simulink model "qddot"  (R2019b)
settings: Solver=ode3  StartTime=0.0  StopTime=10  FixedStep=0.001  RelTol=1e-3  EnableMultiTasking=on
settings Model: ExtModeTrigDuration=5000  Creator=sfukamachi  LastModifiedBy=Chris
settings SolverCC: PositivePriorityOrder=on
settings DataIOCC: LimitDataPoints=on  SaveFormat=Array  ReturnWorkspaceOutputs=off
settings OptimizationCC: ExpressionDepthLimit=2147483647  LifeSpan=inf
settings DebuggingCC: UnderspecifiedInitializationDetection=Classic  MergeDetectMultiDrivingBlocksExec=none  SolverPrmCheckMsg=warning  StateNameClashWarn=warning  SFUnexpectedBacktrackingDiag=warning  SFNoUnconditionalDefaultTransitionDiag=warning  SFExecutionAtInitializationDiag=none  ArithmeticOperatorsInVariantConditions=warning
settings HardwareCC: ProdBitPerPointer=32  ProdBitPerSizeT=32  ProdBitPerPtrDiffT=32  ProdLargestAtomicFloat=None  ProdIntDivRoundTo=Undefined  ProdEndianess=Unspecified  ProdWordSize=32  ProdHWDeviceType=32-bit Generic
settings ModelReferenceCC: PropagateSignalLabelsOutOfModel=off
settings SFSimCC: SimUseLocalCustomCode=off  CustomCodeUndefinedFunction=UseInterfaceOnly
settings RTWCC: Description=QUARC Win64 Target  SystemTargetFile=quarc_win64.tlc  TemplateMakefile=quarc_default_tmf  RTWUseLocalCustomCode=off
settings CodeAppCC: StateflowObjectComments=on
settings STFCustomTargetCC: TargetPreCompLibLocation=C:\PROGRA~3\QUARC\lib\2012b\win64\release  GeneratePreprocessorConditionals=Disable all  CombineOutputUpdateFcns=on  CPPClassGenCompliant=on  SystemTargetFile=quarc_win64.tlc
settings GRTTargetCC: TargetPreCompLibLocation=C:\PROGRA~3\QUARC\lib\2012b\win64\release  TargetLangStandard=C89/C90 (ANSI)  ParMdlRefBuildCompliant=off  CompOptLevelCompliant=off  ConcurrentExecutionCompliant=off  GeneratePreprocessorConditionals=Disable all  MatFileLogging=off  UseToolchainInfoCompliant=off  ExtMode=on  ExtModeMexFile=quarc_comm
settings ConfigComp: CovMetricSettings=dw  CovHtmlReporting=on  CovSaveCumulativeToWorkspaceVar=on  CovSaveSingleToWorkspaceVar=on  CovExternalEMLEnable=off

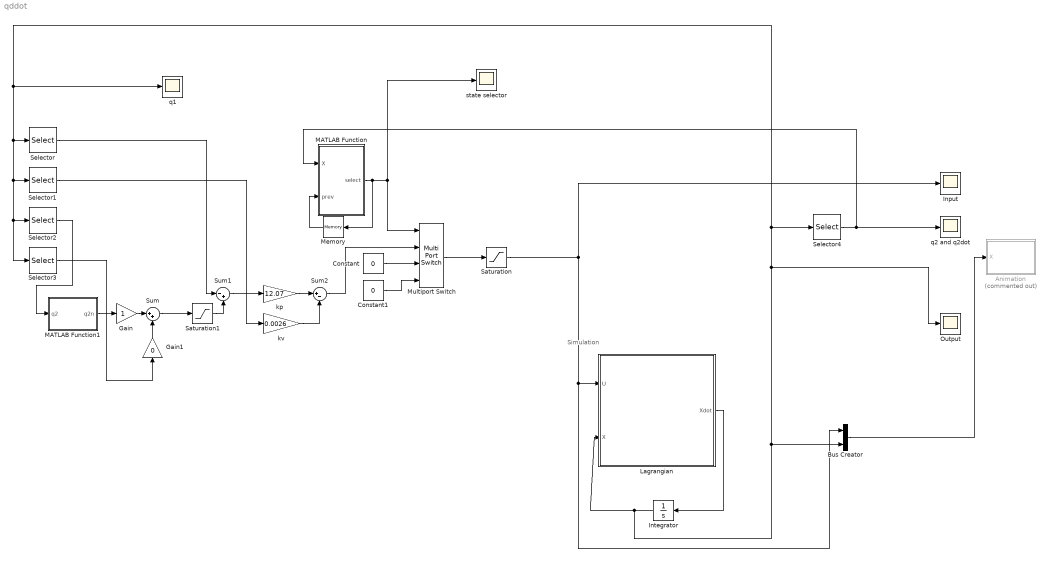
== system qddot ==
  note: Simulation
  Animation : MATLAB Function  Commented=on  TreatAsAtomicUnit=on
  Bus Creator : BusCreator  Inputs=2
  Constant : Constant  Value=0
  Constant1 : Constant  Value=0
  Gain : Gain
  Gain1 : Gain  Gain=0
  Input : Scope
  Integrator : Integrator  InitialCondition=[0; 0; pi; 0]
  Lagrangian : MATLAB Function  TreatAsAtomicUnit=on
  MATLAB Function : MATLAB Function  TreatAsAtomicUnit=on
  MATLAB Function1 : MATLAB Function  TreatAsAtomicUnit=on
  Memory : Memory
  Multiport Switch : MultiPortSwitch
  Output : Scope
  Saturation : Saturate  UpperLimit=10  LowerLimit=-10
  Saturation1 : Saturate  UpperLimit=pi/6  LowerLimit=-pi/6
  Selector : Selector  InputPortWidth=4  IndexOptions=Index vector (dialog)  Indices=[1]  OutputSizes=1
  Selector1 : Selector  InputPortWidth=4  IndexOptions=Index vector (dialog)  Indices=[2]  OutputSizes=1
  Selector2 : Selector  InputPortWidth=4  IndexOptions=Index vector (dialog)  Indices=[3]  OutputSizes=1
  Selector3 : Selector  InputPortWidth=4  IndexOptions=Index vector (dialog)  Indices=[4]  OutputSizes=1
  Selector4 : Selector  InputPortWidth=4  IndexOptions=Index vector (dialog)  Indices=[3 4]  OutputSizes=1
  Sum : Sum  Inputs=|++
  Sum1 : Sum  Inputs=|-+
  Sum2 : Sum  Inputs=|+-
  kp : Gain  Gain=12.07
  kv : Gain  Gain=0.0026
  "q1 " : Scope
  q2 and q2dot : Scope
  state selector : Scope
  wires:
  Saturation/1 -> Bus Creator/1, Lagrangian/1(U), Input/1
  Multiport Switch/1 -> Saturation/1
  Constant/1 -> Multiport Switch/3
  Constant1/1 -> Multiport Switch/4
  Sum2/1 -> Multiport Switch/2
  MATLAB Function/1(select) -> Memory/1, Multiport Switch/1, state selector/1
  Memory/1 -> MATLAB Function/2(prev)
  MATLAB Function1/1(q2n) -> Gain/1
  Gain/1 -> Sum/1
  Gain1/1 -> Sum/2
  Sum/1 -> Saturation1/1
  Saturation1/1 -> Sum1/2
  Sum1/1 -> kp/1
  kp/1 -> Sum2/1
  kv/1 -> Sum2/2
  Bus Creator/1 -> Animation/1(X)
  Lagrangian/1(Xdot) -> Integrator/1
  Selector/1 -> Sum1/1
  Selector1/1 -> kv/1
  Selector2/1 -> MATLAB Function1/1(q2)
  Selector3/1 -> Gain1/1
  Selector4/1 -> q2 and q2dot/1, MATLAB Function/1(X)
  Integrator/1 -> Selector4/1, "q1 "/1, Selector3/1, Selector2/1, Selector1/1, Selector/1, Output/1, Bus Creator/2, Lagrangian/2(X)

== matlab function qddot/Animation ==
  data: X input
function Simulation(X)
Link2P1 = [0;0;0;];
Link2P2 = [0;12;0;];
FRAME2Des = [Link2P1,Link2P2];

Link1P1 = [0;0;0;];
Link1P2 = [0;0;-1;];
Link1P3 = [0;6;-1;];
Link1P4 = [0;6;0;];
Link1P5 = [0;8;0;];
FRAME1Des = [Link1P1,Link1P2,Link1P3,Link1P4,Link1P5];

BaseP1 = [0;0;-10;];
BaseP2 = [0;0;0;];
FRAME0 = [BaseP1,BaseP2];


FRAME0X = FRAME0(1,:);
FRAME0Y = FRAME0(2,:);
FRAME0Z = FRAME0(3,:);
plot3(FRAME0X,FRAME0Y,FRAME0Z,'rs-');
%axis([-15 15 -15 15 -15 15]);
%grid on
hold on

FRAME1 = TRANS0_1(FRAME1Des,X(1));
FRAME1X=FRAME1(1,:);
FRAME1Y=FRAME1(2,:);
FRAME1Z=FRAME1(3,:);


FRAME02 = TRANS0_2(FRAME2Des,X(1),X(3));
FRAME2X=FRAME02(1,:);
FRAME2Y=FRAME02(2,:);
FRAME2Z=FRAME02(3,:);
plot3(FRAME1X,FRAME1Y,FRAME1Z,'b-');
hold on
plot3(FRAME2X,FRAME2Y,FRAME2Z,'g-');
axis([-15 15 -15 15 -15 15]);
grid on
hold off
end

== matlab function qddot/MATLAB Function ==
  data: X input; select output; prev input
function select = fcn(X,prev)
q2 = X(1);
q2dot = X(2);

q2 = 2*atan2(tan(q2/2),1);

select = 2;

if prev == 2
    if abs(q2dot) <= 0.01
        if abs(q2) > 170*2*pi/360
            select = 1;
        end 
    else
        select = 2;
    end
end
        
if prev == 1
    if abs(q2) < 20*2*pi/360
        select = 3;
    else 
        select = 1;
    end
end

if prev == 3
    if abs(q2) > 20*2*pi/360
        select = 2;
    else 
        select = 3;
    end
end

end

== matlab function qddot/Lagrangian ==
  data: U input; Xdot output; X input
function Xdot = Dynamics(U, X)
J1 = 0.0012;
m2 = 0.127;
L12p = 0.2;
L2 = 0.3;
Lc2 = 0.15;
Beta1 = 0.015;
Beta2 = 0.002;
Ra = 2.6;
kt = 0.00768;
kv = 0.00768;
kr = 70;
g = 9.81;

Theta1p = J1 + m2*(L12p)^2;
Theta2p = (1/3)*m2*(L2)^2;
Theta3p = 0.5*m2*(L12p)*L2;
Theta4p = m2*Lc2;

Theta1 = Theta1p * Ra/(kr*kt);
Theta2 = Theta2p * Ra/(kr*kt);
Theta3 = Theta3p * Ra/(kr*kt);
Theta4 = Theta4p * Ra/(kr*kt);
Theta5 = Beta1 * Ra/(kr*kt) + kr*kv;
Theta6 = Beta2 * Ra/(kr*kt);

% X = zeros(4,1);
% X = [q1; q1dot; q2; q2dot];
% V = [v; 0];
M = [Theta1+Theta2*sin(X(3))^2 Theta3*cos(X(3)); Theta3*cos(X(3)) Theta2];
C = [2*Theta2*sin(X(3))*cos(X(3))*X(4) -Theta3*sin(X(3))*X(4); -Theta2*sin(X(3))*cos(X(3))*X(2) 0];
F = [Theta5*X(2); Theta6*X(4)];
G = [0; -Theta4*g*sin(X(3))];
%qddot = zeros(2,1);
Volt = [U; 0];
qddotresult = inv(M)*(Volt - C*[X(2); X(4)] - F - G);
qddot1 = qddotresult(1);
qddot2 = qddotresult(2);
qddot = [qddot1; qddot2];
%Xdot = zeros(4,1);
Xdot = [X(2); qddot(1); X(4); qddot(2)];
end

== matlab function qddot/MATLAB Function1 ==
  data: q2 input; q2n output
function q2n = fcn(q2)

q2n = atan2(sin(q2-pi),cos(q2-pi));
end
